simulink model "model"  (R2024a)
settings: Solver=VariableStepAuto  StartTime=0.0  StopTime=10.0  RelTol=1e-3
libraries: dspsigops x11, commdigbbndpm3 x1, commrandsrc3 x1, simulink x1
settings Model: Creator=abc  LastModifiedBy=abc

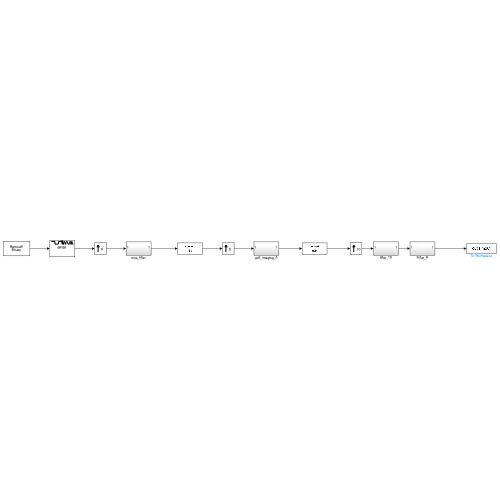
[thumbnail: Simulink's stored preview of the top-level diagram]
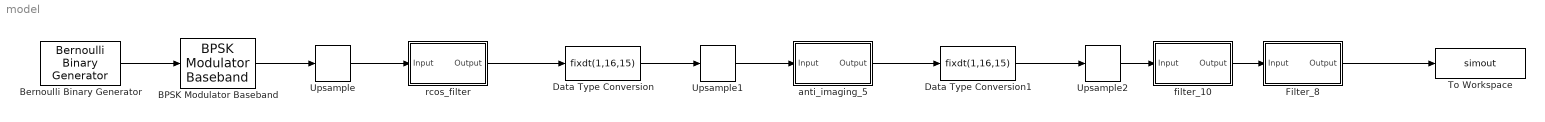
== system model ==
  BPSK Modulator Baseband : commdigbbndpm3/BPSK Modulator Baseband  Ph=0  outDtype=double  outWordLen=16  outUDDataType=sfix(16)  outFracLenMode=Best precision  outFracLen=15  outDataTypeStr=double  outLastDataTypeStr=double
  Bernoulli Binary Generator : commrandsrc3/Bernoulli Binary Generator  ProbabilityOfZero=0.5  SeedSource=Auto  Seed=0  SampleTime=1/400e3  SamplesPerFrame=1  OutputDataType=double  SimulateUsing=Interpreted execution
  Data Type Conversion : DataTypeConversion  OutDataTypeStr=fixdt(1,16,15)  ConvertRealWorld=Stored Integer (SI)  SaturateOnIntegerOverflow=off  RndMeth=Floor
  Data Type Conversion1 : DataTypeConversion  OutDataTypeStr=fixdt(1,16,15)  ConvertRealWorld=Stored Integer (SI)  SaturateOnIntegerOverflow=off  RndMeth=Floor
  Filter_8 : Subsystem  Tag=FilterWizardSubSystem
      settings: ErrorFcn=dspFilterRealizedInBasicElemsAlgLoopErrFcnCallback
  To Workspace : ToWorkspace  VariableName=simout  SampleTime=-1
      settings: Save2DSignal=2-D array (concatenate along first dimension)
  Upsample : dspsigops/Upsample  FactorSource=Dialog parameter  N=9  Nmax=16  phase=0  RateOptions=Allow multirate processing  ic=0  mode=Unused parameter value
  Upsample1 : dspsigops/Upsample  FactorSource=Dialog parameter  N=5  Nmax=16  phase=0  RateOptions=Allow multirate processing  ic=0  mode=Unused parameter value
  Upsample2 : dspsigops/Upsample  FactorSource=Dialog parameter  N=10  Nmax=16  phase=0  RateOptions=Allow multirate processing  ic=0  mode=Unused parameter value
  anti_imaging_5 : Subsystem  Tag=FilterWizardSubSystem
      settings: ErrorFcn=dspFilterRealizedInBasicElemsAlgLoopErrFcnCallback
  filter_10 : Subsystem  Tag=FilterWizardSubSystem
      settings: ErrorFcn=dspFilterRealizedInBasicElemsAlgLoopErrFcnCallback
  rcos_filter : Subsystem  Tag=FilterWizardSubSystem
      settings: ErrorFcn=dspFilterRealizedInBasicElemsAlgLoopErrFcnCallback
  wires:
  Bernoulli Binary Generator/1 -> BPSK Modulator Baseband/1
  BPSK Modulator Baseband/1 -> Upsample/1
  Upsample/1 -> rcos_filter/1(Input)
  rcos_filter/1(Output) -> Data Type Conversion/1
  Data Type Conversion/1 -> Upsample1/1
  Upsample1/1 -> anti_imaging_5/1(Input)
  anti_imaging_5/1(Output) -> Data Type Conversion1/1
  Data Type Conversion1/1 -> Upsample2/1
  Upsample2/1 -> filter_10/1(Input)
  filter_10/1(Output) -> Filter_8/1(Input)
  Filter_8/1(Output) -> To Workspace/1

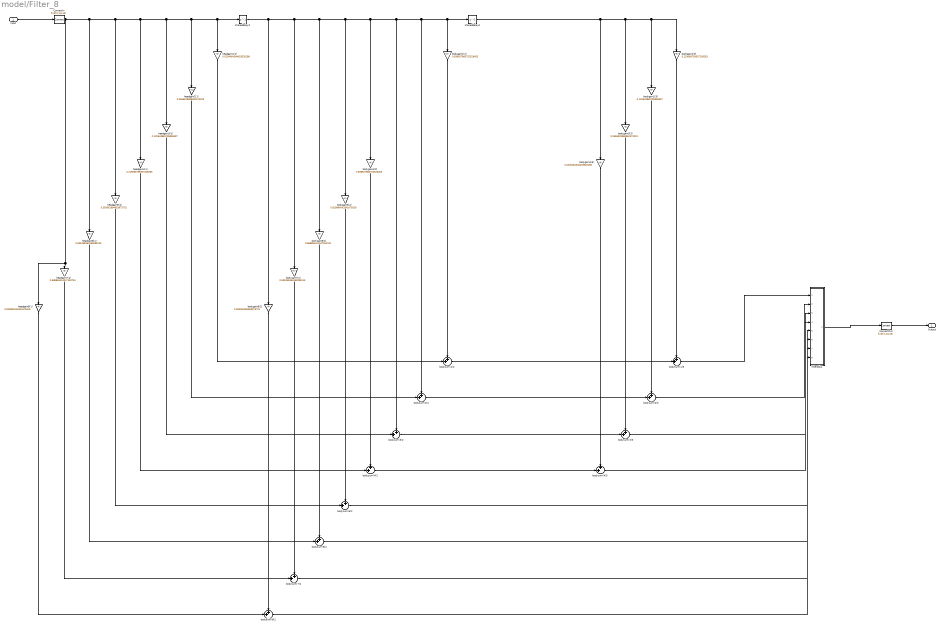
== system model/Filter_8 ==
  Input : Inport
  ConvertIn : DataTypeConversion  OutDataTypeStr=fixdt(1,16,15)  RndMeth=Nearest
  ConvertOut : DataTypeConversion  OutDataTypeStr=fixdt(1,16,15)  RndMeth=Convergent  SaturateOnIntegerOverflow=off
  InterpSys : Subsystem  Tag=FilterWizardInterpolatorCommutator
  bodygain1(2) : Gain  Gain=0.936507860752529453  ParamDataTypeStr=fixdt(1,16,15)  OutDataTypeStr=fixdt(1,31,30)  RndMeth=Convergent
  bodygain1(3) : Gain  Gain=0.219069759307206263  ParamDataTypeStr=fixdt(1,16,15)  OutDataTypeStr=fixdt(1,31,30)  RndMeth=Convergent
  bodygain2(3) : Gain  Gain=0.120643855795995597  ParamDataTypeStr=fixdt(1,16,15)  OutDataTypeStr=fixdt(1,31,30)  RndMeth=Convergent
  bodygain3(3) : Gain  Gain=0.0556329388362373223  ParamDataTypeStr=fixdt(1,16,15)  OutDataTypeStr=fixdt(1,31,30)  RndMeth=Convergent
  bodygain4(2) : Gain  Gain=0.936507860752529453  ParamDataTypeStr=fixdt(1,16,15)  OutDataTypeStr=fixdt(1,31,30)  RndMeth=Convergent
  bodygain4(3) : Gain  Gain=0.0200464348433526188  ParamDataTypeStr=fixdt(1,16,15)  OutDataTypeStr=fixdt(1,31,30)  RndMeth=Convergent
  bodygain5(2) : Gain  Gain=0.819994042841679316  ParamDataTypeStr=fixdt(1,16,15)  OutDataTypeStr=fixdt(1,31,30)  RndMeth=Convergent
  bodygain6(2) : Gain  Gain=0.668884424047150761  ParamDataTypeStr=fixdt(1,16,15)  OutDataTypeStr=fixdt(1,31,30)  RndMeth=Convergent
  bodygain7(2) : Gain  Gain=0.505255361559098115  ParamDataTypeStr=fixdt(1,16,15)  OutDataTypeStr=fixdt(1,31,30)  RndMeth=Convergent
  bodygain8(2) : Gain  Gain=0.350061984653973701  ParamDataTypeStr=fixdt(1,16,15)  OutDataTypeStr=fixdt(1,31,30)  RndMeth=Convergent
  bodysum(1)2 : Sum  Inputs=++|  OutDataTypeStr=fixdt(1,32,30)  AccumDataTypeStr=fixdt(1,32,30)  RndMeth=Convergent
  bodysum(1)3 : Sum  Inputs=++|  OutDataTypeStr=fixdt(1,32,30)  AccumDataTypeStr=fixdt(1,32,30)  RndMeth=Convergent
  bodysum(2)2 : Sum  Inputs=++|  OutDataTypeStr=fixdt(1,32,30)  AccumDataTypeStr=fixdt(1,32,30)  RndMeth=Convergent
  bodysum(2)3 : Sum  Inputs=++|  OutDataTypeStr=fixdt(1,32,30)  AccumDataTypeStr=fixdt(1,32,30)  RndMeth=Convergent
  bodysum(3)2 : Sum  Inputs=++|  OutDataTypeStr=fixdt(1,32,30)  AccumDataTypeStr=fixdt(1,32,30)  RndMeth=Convergent
  bodysum(3)3 : Sum  Inputs=++|  OutDataTypeStr=fixdt(1,32,30)  AccumDataTypeStr=fixdt(1,32,30)  RndMeth=Convergent
  bodysum(4)2 : Sum  Inputs=++|  OutDataTypeStr=fixdt(1,32,30)  AccumDataTypeStr=fixdt(1,32,30)  RndMeth=Convergent
  bodysum(4)3 : Sum  Inputs=++|  OutDataTypeStr=fixdt(1,32,30)  AccumDataTypeStr=fixdt(1,32,30)  RndMeth=Convergent
  bodysum(5)2 : Sum  Inputs=++|  OutDataTypeStr=fixdt(1,32,30)  AccumDataTypeStr=fixdt(1,32,30)  RndMeth=Convergent
  bodysum(6)2 : Sum  Inputs=++|  OutDataTypeStr=fixdt(1,32,30)  AccumDataTypeStr=fixdt(1,32,30)  RndMeth=Convergent
  bodysum(7)2 : Sum  Inputs=++|  OutDataTypeStr=fixdt(1,32,30)  AccumDataTypeStr=fixdt(1,32,30)  RndMeth=Convergent
  bodysum(8)2 : Sum  Inputs=++|  OutDataTypeStr=fixdt(1,32,30)  AccumDataTypeStr=fixdt(1,32,30)  RndMeth=Convergent
  headgain1(1) : Gain  Gain=0.0200464348433526188  ParamDataTypeStr=fixdt(1,16,15)  OutDataTypeStr=fixdt(1,31,30)  RndMeth=Convergent
  headgain2(1) : Gain  Gain=0.0556329388362373223  ParamDataTypeStr=fixdt(1,16,15)  OutDataTypeStr=fixdt(1,31,30)  RndMeth=Convergent
  headgain3(1) : Gain  Gain=0.120643855795995597  ParamDataTypeStr=fixdt(1,16,15)  OutDataTypeStr=fixdt(1,31,30)  RndMeth=Convergent
  headgain4(1) : Gain  Gain=0.219069759307206263  ParamDataTypeStr=fixdt(1,16,15)  OutDataTypeStr=fixdt(1,31,30)  RndMeth=Convergent
  headgain5(1) : Gain  Gain=0.350061984653973701  ParamDataTypeStr=fixdt(1,16,15)  OutDataTypeStr=fixdt(1,31,30)  RndMeth=Convergent
  headgain6(1) : Gain  Gain=0.505255361559098115  ParamDataTypeStr=fixdt(1,16,15)  OutDataTypeStr=fixdt(1,31,30)  RndMeth=Convergent
  headgain7(1) : Gain  Gain=0.668884424047150761  ParamDataTypeStr=fixdt(1,16,15)  OutDataTypeStr=fixdt(1,31,30)  RndMeth=Convergent
  headgain8(1) : Gain  Gain=0.819994042841679316  ParamDataTypeStr=fixdt(1,16,15)  OutDataTypeStr=fixdt(1,31,30)  RndMeth=Convergent
  shareddelay2 : Delay  DelayLength=1  InitialCondition=0
  shareddelay3 : Delay  DelayLength=1  InitialCondition=0
  Output : Outport
  wires:
  headgain1(1)/1 -> bodysum(1)2/2
  headgain2(1)/1 -> bodysum(2)2/2
  headgain3(1)/1 -> bodysum(3)2/2
  headgain4(1)/1 -> bodysum(4)2/2
  headgain5(1)/1 -> bodysum(5)2/2
  headgain6(1)/1 -> bodysum(6)2/2
  headgain7(1)/1 -> bodysum(7)2/2
  headgain8(1)/1 -> bodysum(8)2/2
  Input/1 -> ConvertIn/1
  ConvertIn/1 -> headgain7(1)/1, headgain8(1)/1, headgain1(1)/1, shareddelay2/1, headgain2(1)/1, headgain3(1)/1, headgain4(1)/1, headgain5(1)/1, headgain6(1)/1
  bodygain1(2)/1 -> bodysum(1)2/1
  bodygain4(2)/1 -> bodysum(4)2/1
  bodygain5(2)/1 -> bodysum(5)2/1
  bodygain6(2)/1 -> bodysum(6)2/1
  bodygain7(2)/1 -> bodysum(7)2/1
  bodygain8(2)/1 -> bodysum(8)2/1
  bodysum(1)2/1 -> bodysum(1)3/2
  bodysum(2)2/1 -> bodysum(2)3/2
  bodysum(3)2/1 -> bodysum(3)3/2
  bodysum(4)2/1 -> bodysum(4)3/2
  bodysum(5)2/1 -> InterpSys/5(input5)
  bodysum(6)2/1 -> InterpSys/6(input6)
  bodysum(7)2/1 -> InterpSys/7(input7)
  bodysum(8)2/1 -> InterpSys/8(input8)
  shareddelay2/1 -> bodygain1(2)/1, shareddelay3/1, bodysum(2)2/1, bodysum(3)2/1, bodygain4(2)/1, bodygain5(2)/1, bodygain6(2)/1, bodygain7(2)/1, bodygain8(2)/1
  bodygain1(3)/1 -> bodysum(1)3/1
  bodygain2(3)/1 -> bodysum(2)3/1
  bodygain3(3)/1 -> bodysum(3)3/1
  bodygain4(3)/1 -> bodysum(4)3/1
  bodysum(1)3/1 -> InterpSys/1(input1)
  bodysum(2)3/1 -> InterpSys/2(input2)
  bodysum(3)3/1 -> InterpSys/3(input3)
  bodysum(4)3/1 -> InterpSys/4(input4)
  shareddelay3/1 -> bodygain1(3)/1, bodygain2(3)/1, bodygain3(3)/1, bodygain4(3)/1
  InterpSys/1(output) -> ConvertOut/1
  ConvertOut/1 -> Output/1

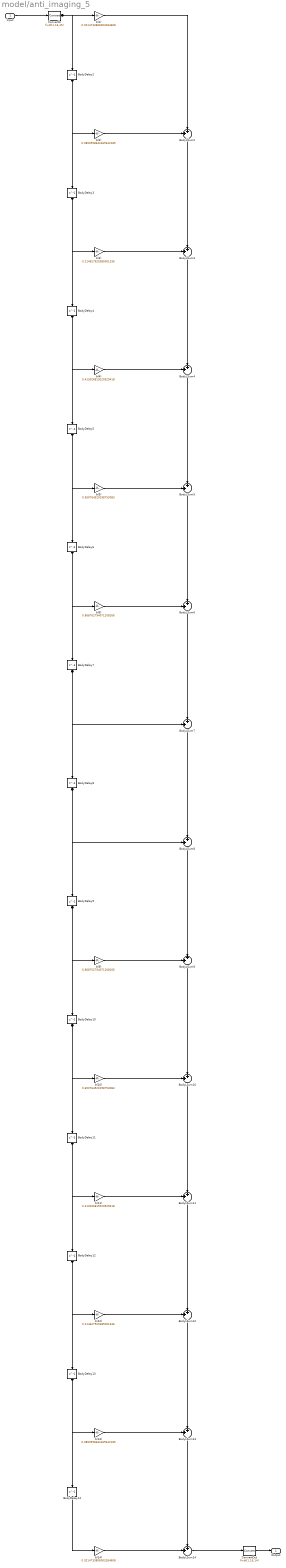
== system model/anti_imaging_5 ==
  Input : Inport
  BodyDelay{2..14} (13 alike) : Delay  DelayLength=1  InitialCondition=0
  BodyLSum{2..14} (13 alike) : Sum  Inputs=++|  OutDataTypeStr=fixdt(1,33,29)  AccumDataTypeStr=fixdt(1,33,29)  RndMeth=Convergent
  ConvertIn : DataTypeConversion  OutDataTypeStr=fixdt(1,16,15)  RndMeth=Nearest
  ConvertOut : DataTypeConversion  OutDataTypeStr=fixdt(1,16,14)  RndMeth=Convergent  SaturateOnIntegerOverflow=off
  b(1) : Gain  Gain=0.0214733806003284608  ParamDataTypeStr=fixdt(1,16,14)  OutDataTypeStr=fixdt(1,31,29)  RndMeth=Convergent
  b(10) : Gain  Gain=0.650764520198753083  ParamDataTypeStr=fixdt(1,16,14)  OutDataTypeStr=fixdt(1,31,29)  RndMeth=Convergent
  b(11) : Gain  Gain=0.413026819220529418  ParamDataTypeStr=fixdt(1,16,14)  OutDataTypeStr=fixdt(1,31,29)  RndMeth=Convergent
  b(12) : Gain  Gain=0.214627920385001336  ParamDataTypeStr=fixdt(1,16,14)  OutDataTypeStr=fixdt(1,31,29)  RndMeth=Convergent
  b(13) : Gain  Gain=0.0850558632469342185  ParamDataTypeStr=fixdt(1,16,14)  OutDataTypeStr=fixdt(1,31,29)  RndMeth=Convergent
  b(14) : Gain  Gain=0.0214733806003284608  ParamDataTypeStr=fixdt(1,16,14)  OutDataTypeStr=fixdt(1,31,29)  RndMeth=Convergent
  b(2) : Gain  Gain=0.0850558632469342185  ParamDataTypeStr=fixdt(1,16,14)  OutDataTypeStr=fixdt(1,31,29)  RndMeth=Convergent
  b(3) : Gain  Gain=0.214627920385001336  ParamDataTypeStr=fixdt(1,16,14)  OutDataTypeStr=fixdt(1,31,29)  RndMeth=Convergent
  b(4) : Gain  Gain=0.413026819220529418  ParamDataTypeStr=fixdt(1,16,14)  OutDataTypeStr=fixdt(1,31,29)  RndMeth=Convergent
  b(5) : Gain  Gain=0.650764520198753083  ParamDataTypeStr=fixdt(1,16,14)  OutDataTypeStr=fixdt(1,31,29)  RndMeth=Convergent
  b(6) : Gain  Gain=0.868762794071208266  ParamDataTypeStr=fixdt(1,16,14)  OutDataTypeStr=fixdt(1,31,29)  RndMeth=Convergent
  b(9) : Gain  Gain=0.868762794071208266  ParamDataTypeStr=fixdt(1,16,14)  OutDataTypeStr=fixdt(1,31,29)  RndMeth=Convergent
  Output : Outport
  wires:
  Input/1 -> ConvertIn/1
  b(1)/1 -> BodyLSum2/2
  ConvertIn/1 -> b(1)/1, BodyDelay2/1
  BodyDelay2/1 -> b(2)/1, BodyDelay3/1
  b(2)/1 -> BodyLSum2/1
  BodyLSum2/1 -> BodyLSum3/2
  BodyDelay3/1 -> b(3)/1, BodyDelay4/1
  b(3)/1 -> BodyLSum3/1
  BodyLSum3/1 -> BodyLSum4/2
  BodyDelay4/1 -> b(4)/1, BodyDelay5/1
  b(4)/1 -> BodyLSum4/1
  BodyLSum4/1 -> BodyLSum5/2
  BodyDelay5/1 -> b(5)/1, BodyDelay6/1
  b(5)/1 -> BodyLSum5/1
  BodyLSum5/1 -> BodyLSum6/2
  BodyDelay6/1 -> b(6)/1, BodyDelay7/1
  b(6)/1 -> BodyLSum6/1
  BodyLSum6/1 -> BodyLSum7/2
  BodyDelay7/1 -> BodyLSum7/1, BodyDelay8/1
  BodyLSum7/1 -> BodyLSum8/2
  BodyDelay8/1 -> BodyLSum8/1, BodyDelay9/1
  BodyLSum8/1 -> BodyLSum9/2
  BodyDelay9/1 -> b(9)/1, BodyDelay10/1
  b(9)/1 -> BodyLSum9/1
  BodyLSum9/1 -> BodyLSum10/2
  BodyDelay10/1 -> b(10)/1, BodyDelay11/1
  b(10)/1 -> BodyLSum10/1
  BodyLSum10/1 -> BodyLSum11/2
  BodyDelay11/1 -> b(11)/1, BodyDelay12/1
  b(11)/1 -> BodyLSum11/1
  BodyLSum11/1 -> BodyLSum12/2
  BodyDelay12/1 -> b(12)/1, BodyDelay13/1
  b(12)/1 -> BodyLSum12/1
  BodyLSum12/1 -> BodyLSum13/2
  BodyDelay13/1 -> b(13)/1, BodyDelay14/1
  b(13)/1 -> BodyLSum13/1
  BodyLSum13/1 -> BodyLSum14/1
  BodyDelay14/1 -> b(14)/1
  b(14)/1 -> BodyLSum14/2
  BodyLSum14/1 -> ConvertOut/1
  ConvertOut/1 -> Output/1

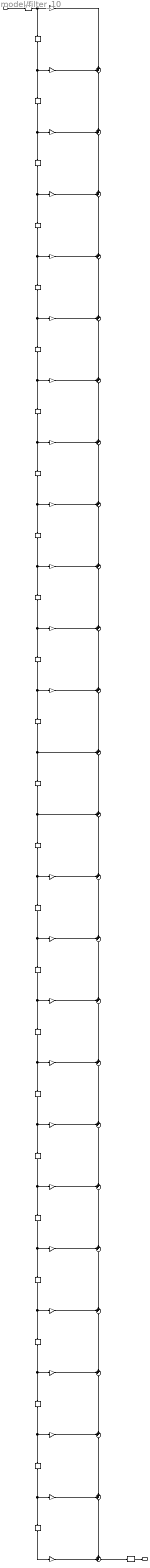
== system model/filter_10 ==
  Input : Inport
  BodyDelay{2..26} (25 alike) : Delay  DelayLength=1  InitialCondition=0
  BodyLSum{2..26} (25 alike) : Sum  Inputs=++|  OutDataTypeStr=fixdt(1,35,30)  AccumDataTypeStr=fixdt(1,35,30)  RndMeth=Convergent
  ConvertIn : DataTypeConversion  OutDataTypeStr=fixdt(1,16,15)  RndMeth=Nearest
  ConvertOut : DataTypeConversion  OutDataTypeStr=fixdt(1,16,15)  RndMeth=Convergent  SaturateOnIntegerOverflow=off
  b(1) : Gain  Gain=0.0154934539007253128  ParamDataTypeStr=fixdt(1,16,15)  OutDataTypeStr=fixdt(1,31,30)  RndMeth=Convergent
  b(10) : Gain  Gain=0.784532005187096648  ParamDataTypeStr=fixdt(1,16,15)  OutDataTypeStr=fixdt(1,31,30)  RndMeth=Convergent
  b(11) : Gain  Gain=0.886548728923319596  ParamDataTypeStr=fixdt(1,16,15)  OutDataTypeStr=fixdt(1,31,30)  RndMeth=Convergent
  b(12) : Gain  Gain=0.960846421505135662  ParamDataTypeStr=fixdt(1,16,15)  OutDataTypeStr=fixdt(1,31,30)  RndMeth=Convergent
  b(15) : Gain  Gain=0.960846421505135662  ParamDataTypeStr=fixdt(1,16,15)  OutDataTypeStr=fixdt(1,31,30)  RndMeth=Convergent
  b(16) : Gain  Gain=0.886548728923319596  ParamDataTypeStr=fixdt(1,16,15)  OutDataTypeStr=fixdt(1,31,30)  RndMeth=Convergent
  b(17) : Gain  Gain=0.784532005187096648  ParamDataTypeStr=fixdt(1,16,15)  OutDataTypeStr=fixdt(1,31,30)  RndMeth=Convergent
  b(18) : Gain  Gain=0.664532684409961938  ParamDataTypeStr=fixdt(1,16,15)  OutDataTypeStr=fixdt(1,31,30)  RndMeth=Convergent
  b(19) : Gain  Gain=0.537212909502194136  ParamDataTypeStr=fixdt(1,16,15)  OutDataTypeStr=fixdt(1,31,30)  RndMeth=Convergent
  b(2) : Gain  Gain=0.0360061265388371618  ParamDataTypeStr=fixdt(1,16,15)  OutDataTypeStr=fixdt(1,31,30)  RndMeth=Convergent
  b(20) : Gain  Gain=0.412761582748364442  ParamDataTypeStr=fixdt(1,16,15)  OutDataTypeStr=fixdt(1,31,30)  RndMeth=Convergent
  b(21) : Gain  Gain=0.299634419816256437  ParamDataTypeStr=fixdt(1,16,15)  OutDataTypeStr=fixdt(1,31,30)  RndMeth=Convergent
  b(22) : Gain  Gain=0.203733323531139293  ParamDataTypeStr=fixdt(1,16,15)  OutDataTypeStr=fixdt(1,31,30)  RndMeth=Convergent
  b(23) : Gain  Gain=0.128056316959141631  ParamDataTypeStr=fixdt(1,16,15)  OutDataTypeStr=fixdt(1,31,30)  RndMeth=Convergent
  b(24) : Gain  Gain=0.0728175851807882912  ParamDataTypeStr=fixdt(1,16,15)  OutDataTypeStr=fixdt(1,31,30)  RndMeth=Convergent
  b(25) : Gain  Gain=0.0360061265388371618  ParamDataTypeStr=fixdt(1,16,15)  OutDataTypeStr=fixdt(1,31,30)  RndMeth=Convergent
  b(26) : Gain  Gain=0.0154934539007253128  ParamDataTypeStr=fixdt(1,16,15)  OutDataTypeStr=fixdt(1,31,30)  RndMeth=Convergent
  b(3) : Gain  Gain=0.0728175851807882912  ParamDataTypeStr=fixdt(1,16,15)  OutDataTypeStr=fixdt(1,31,30)  RndMeth=Convergent
  b(4) : Gain  Gain=0.128056316959141631  ParamDataTypeStr=fixdt(1,16,15)  OutDataTypeStr=fixdt(1,31,30)  RndMeth=Convergent
  b(5) : Gain  Gain=0.203733323531139293  ParamDataTypeStr=fixdt(1,16,15)  OutDataTypeStr=fixdt(1,31,30)  RndMeth=Convergent
  b(6) : Gain  Gain=0.299634419816256437  ParamDataTypeStr=fixdt(1,16,15)  OutDataTypeStr=fixdt(1,31,30)  RndMeth=Convergent
  b(7) : Gain  Gain=0.412761582748364442  ParamDataTypeStr=fixdt(1,16,15)  OutDataTypeStr=fixdt(1,31,30)  RndMeth=Convergent
  b(8) : Gain  Gain=0.537212909502194136  ParamDataTypeStr=fixdt(1,16,15)  OutDataTypeStr=fixdt(1,31,30)  RndMeth=Convergent
  b(9) : Gain  Gain=0.664532684409961938  ParamDataTypeStr=fixdt(1,16,15)  OutDataTypeStr=fixdt(1,31,30)  RndMeth=Convergent
  Output : Outport
  wires:
  Input/1 -> ConvertIn/1
  b(1)/1 -> BodyLSum2/2
  ConvertIn/1 -> b(1)/1, BodyDelay2/1
  BodyDelay2/1 -> b(2)/1, BodyDelay3/1
  b(2)/1 -> BodyLSum2/1
  BodyLSum2/1 -> BodyLSum3/2
  BodyDelay3/1 -> b(3)/1, BodyDelay4/1
  b(3)/1 -> BodyLSum3/1
  BodyLSum3/1 -> BodyLSum4/2
  BodyDelay4/1 -> b(4)/1, BodyDelay5/1
  b(4)/1 -> BodyLSum4/1
  BodyLSum4/1 -> BodyLSum5/2
  BodyDelay5/1 -> b(5)/1, BodyDelay6/1
  b(5)/1 -> BodyLSum5/1
  BodyLSum5/1 -> BodyLSum6/2
  BodyDelay6/1 -> b(6)/1, BodyDelay7/1
  b(6)/1 -> BodyLSum6/1
  BodyLSum6/1 -> BodyLSum7/2
  BodyDelay7/1 -> b(7)/1, BodyDelay8/1
  b(7)/1 -> BodyLSum7/1
  BodyLSum7/1 -> BodyLSum8/2
  BodyDelay8/1 -> b(8)/1, BodyDelay9/1
  b(8)/1 -> BodyLSum8/1
  BodyLSum8/1 -> BodyLSum9/2
  BodyDelay9/1 -> b(9)/1, BodyDelay10/1
  b(9)/1 -> BodyLSum9/1
  BodyLSum9/1 -> BodyLSum10/2
  BodyDelay10/1 -> b(10)/1, BodyDelay11/1
  b(10)/1 -> BodyLSum10/1
  BodyLSum10/1 -> BodyLSum11/2
  BodyDelay11/1 -> b(11)/1, BodyDelay12/1
  b(11)/1 -> BodyLSum11/1
  BodyLSum11/1 -> BodyLSum12/2
  BodyDelay12/1 -> b(12)/1, BodyDelay13/1
  b(12)/1 -> BodyLSum12/1
  BodyLSum12/1 -> BodyLSum13/2
  BodyDelay13/1 -> BodyLSum13/1, BodyDelay14/1
  BodyLSum13/1 -> BodyLSum14/2
  BodyDelay14/1 -> BodyLSum14/1, BodyDelay15/1
  BodyLSum14/1 -> BodyLSum15/2
  BodyDelay15/1 -> b(15)/1, BodyDelay16/1
  b(15)/1 -> BodyLSum15/1
  BodyLSum15/1 -> BodyLSum16/2
  BodyDelay16/1 -> b(16)/1, BodyDelay17/1
  b(16)/1 -> BodyLSum16/1
  BodyLSum16/1 -> BodyLSum17/2
  BodyDelay17/1 -> b(17)/1, BodyDelay18/1
  b(17)/1 -> BodyLSum17/1
  BodyLSum17/1 -> BodyLSum18/2
  BodyDelay18/1 -> b(18)/1, BodyDelay19/1
  b(18)/1 -> BodyLSum18/1
  BodyLSum18/1 -> BodyLSum19/2
  BodyDelay19/1 -> b(19)/1, BodyDelay20/1
  b(19)/1 -> BodyLSum19/1
  BodyLSum19/1 -> BodyLSum20/2
  BodyDelay20/1 -> b(20)/1, BodyDelay21/1
  b(20)/1 -> BodyLSum20/1
  BodyLSum20/1 -> BodyLSum21/2
  BodyDelay21/1 -> b(21)/1, BodyDelay22/1
  b(21)/1 -> BodyLSum21/1
  BodyLSum21/1 -> BodyLSum22/2
  BodyDelay22/1 -> b(22)/1, BodyDelay23/1
  b(22)/1 -> BodyLSum22/1
  BodyLSum22/1 -> BodyLSum23/2
  BodyDelay23/1 -> b(23)/1, BodyDelay24/1
  b(23)/1 -> BodyLSum23/1
  BodyLSum23/1 -> BodyLSum24/2
  BodyDelay24/1 -> b(24)/1, BodyDelay25/1
  b(24)/1 -> BodyLSum24/1
  BodyLSum24/1 -> BodyLSum25/2
  BodyDelay25/1 -> b(25)/1, BodyDelay26/1
  b(25)/1 -> BodyLSum25/1
  BodyLSum25/1 -> BodyLSum26/1
  BodyDelay26/1 -> b(26)/1
  b(26)/1 -> BodyLSum26/2
  BodyLSum26/1 -> ConvertOut/1
  ConvertOut/1 -> Output/1

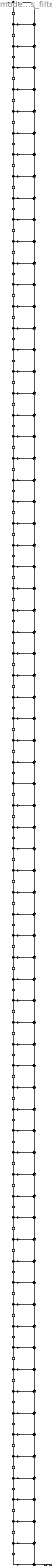
== system model/rcos_filter ==
  Input : Inport
  BodyDelay{2..73} (72 alike) : Delay  DelayLength=1  InitialCondition=0
  BodyLSum{2..73} (72 alike) : Sum  Inputs=++|  OutDataTypeStr=fixdt(1,35,30)  AccumDataTypeStr=fixdt(1,35,30)  RndMeth=Convergent
  ConvertIn : DataTypeConversion  OutDataTypeStr=fixdt(1,16,15)  RndMeth=Nearest
  ConvertOut : DataTypeConversion  OutDataTypeStr=fixdt(1,16,14)  RndMeth=Convergent  SaturateOnIntegerOverflow=off
  b(1) : Gain  Gain=-1.22182503891341904e-17  ParamDataTypeStr=fixdt(1,16,15)  OutDataTypeStr=fixdt(1,31,30)  RndMeth=Convergent
  b(10) : Gain  Gain=2.13059203422986562e-17  ParamDataTypeStr=fixdt(1,16,15)  OutDataTypeStr=fixdt(1,31,30)  RndMeth=Convergent
  b(11) : Gain  Gain=0.021597306460504704  ParamDataTypeStr=fixdt(1,16,15)  OutDataTypeStr=fixdt(1,31,30)  RndMeth=Convergent
  b(12) : Gain  Gain=0.0441571027538437549  ParamDataTypeStr=fixdt(1,16,15)  OutDataTypeStr=fixdt(1,31,30)  RndMeth=Convergent
  b(13) : Gain  Gain=0.0646765061723711676  ParamDataTypeStr=fixdt(1,16,15)  OutDataTypeStr=fixdt(1,31,30)  RndMeth=Convergent
  b(14) : Gain  Gain=0.0799176768301118612  ParamDataTypeStr=fixdt(1,16,15)  OutDataTypeStr=fixdt(1,31,30)  RndMeth=Convergent
  b(15) : Gain  Gain=0.0868181027365576841  ParamDataTypeStr=fixdt(1,16,15)  OutDataTypeStr=fixdt(1,31,30)  RndMeth=Convergent
  b(16) : Gain  Gain=0.0829381759888999509  ParamDataTypeStr=fixdt(1,16,15)  OutDataTypeStr=fixdt(1,31,30)  RndMeth=Convergent
  b(17) : Gain  Gain=0.0668910455890105449  ParamDataTypeStr=fixdt(1,16,15)  OutDataTypeStr=fixdt(1,31,30)  RndMeth=Convergent
  b(18) : Gain  Gain=0.0386959499791306588  ParamDataTypeStr=fixdt(1,16,15)  OutDataTypeStr=fixdt(1,31,30)  RndMeth=Convergent
  b(19) : Gain  Gain=-3.01539353071549505e-17  ParamDataTypeStr=fixdt(1,16,15)  OutDataTypeStr=fixdt(1,31,30)  RndMeth=Convergent
  b(2) : Gain  Gain=-0.00946227947059827962  ParamDataTypeStr=fixdt(1,16,15)  OutDataTypeStr=fixdt(1,31,30)  RndMeth=Convergent
  b(20) : Gain  Gain=-0.0458751609436186536  ParamDataTypeStr=fixdt(1,16,15)  OutDataTypeStr=fixdt(1,31,30)  RndMeth=Convergent
  b(21) : Gain  Gain=-0.0940871562496050223  ParamDataTypeStr=fixdt(1,16,15)  OutDataTypeStr=fixdt(1,31,30)  RndMeth=Convergent
  b(22) : Gain  Gain=-0.138629354352431816  ParamDataTypeStr=fixdt(1,16,15)  OutDataTypeStr=fixdt(1,31,30)  RndMeth=Convergent
  b(23) : Gain  Gain=-0.172866939748332171  ParamDataTypeStr=fixdt(1,16,15)  OutDataTypeStr=fixdt(1,31,30)  RndMeth=Convergent
  b(24) : Gain  Gain=-0.190205163336895938  ParamDataTypeStr=fixdt(1,16,15)  OutDataTypeStr=fixdt(1,31,30)  RndMeth=Convergent
  b(25) : Gain  Gain=-0.184822244508834388  ParamDataTypeStr=fixdt(1,16,15)  OutDataTypeStr=fixdt(1,31,30)  RndMeth=Convergent
  b(26) : Gain  Gain=-0.152386366623032066  ParamDataTypeStr=fixdt(1,16,15)  OutDataTypeStr=fixdt(1,31,30)  RndMeth=Convergent
  b(27) : Gain  Gain=-0.0906723589187520135  ParamDataTypeStr=fixdt(1,16,15)  OutDataTypeStr=fixdt(1,31,30)  RndMeth=Convergent
  b(28) : Gain  Gain=3.66131944315138439e-17  ParamDataTypeStr=fixdt(1,16,15)  OutDataTypeStr=fixdt(1,31,30)  RndMeth=Convergent
  b(29) : Gain  Gain=0.116567855832702696  ParamDataTypeStr=fixdt(1,16,15)  OutDataTypeStr=fixdt(1,31,30)  RndMeth=Convergent
  b(3) : Gain  Gain=-0.0196630498184133598  ParamDataTypeStr=fixdt(1,16,15)  OutDataTypeStr=fixdt(1,31,30)  RndMeth=Convergent
  b(30) : Gain  Gain=0.253304499230267155  ParamDataTypeStr=fixdt(1,16,15)  OutDataTypeStr=fixdt(1,31,30)  RndMeth=Convergent
  b(31) : Gain  Gain=0.402182813135878947  ParamDataTypeStr=fixdt(1,16,15)  OutDataTypeStr=fixdt(1,31,30)  RndMeth=Convergent
  b(32) : Gain  Gain=0.553497404087329614  ParamDataTypeStr=fixdt(1,16,15)  OutDataTypeStr=fixdt(1,31,30)  RndMeth=Convergent
  b(33) : Gain  Gain=0.696689242667723363  ParamDataTypeStr=fixdt(1,16,15)  OutDataTypeStr=fixdt(1,31,30)  RndMeth=Convergent
  b(34) : Gain  Gain=0.821291614576821427  ParamDataTypeStr=fixdt(1,16,15)  OutDataTypeStr=fixdt(1,31,30)  RndMeth=Convergent
  b(35) : Gain  Gain=0.9178999843072434  ParamDataTypeStr=fixdt(1,16,15)  OutDataTypeStr=fixdt(1,31,30)  RndMeth=Convergent
  b(36) : Gain  Gain=0.979063182750591232  ParamDataTypeStr=fixdt(1,16,15)  OutDataTypeStr=fixdt(1,31,30)  RndMeth=Convergent
  b(38) : Gain  Gain=0.979063182750591232  ParamDataTypeStr=fixdt(1,16,15)  OutDataTypeStr=fixdt(1,31,30)  RndMeth=Convergent
  b(39) : Gain  Gain=0.9178999843072434  ParamDataTypeStr=fixdt(1,16,15)  OutDataTypeStr=fixdt(1,31,30)  RndMeth=Convergent
  b(4) : Gain  Gain=-0.0292099363995702542  ParamDataTypeStr=fixdt(1,16,15)  OutDataTypeStr=fixdt(1,31,30)  RndMeth=Convergent
  b(40) : Gain  Gain=0.821291614576821427  ParamDataTypeStr=fixdt(1,16,15)  OutDataTypeStr=fixdt(1,31,30)  RndMeth=Convergent
  b(41) : Gain  Gain=0.696689242667723363  ParamDataTypeStr=fixdt(1,16,15)  OutDataTypeStr=fixdt(1,31,30)  RndMeth=Convergent
  b(42) : Gain  Gain=0.553497404087329614  ParamDataTypeStr=fixdt(1,16,15)  OutDataTypeStr=fixdt(1,31,30)  RndMeth=Convergent
  b(43) : Gain  Gain=0.402182813135878947  ParamDataTypeStr=fixdt(1,16,15)  OutDataTypeStr=fixdt(1,31,30)  RndMeth=Convergent
  b(44) : Gain  Gain=0.253304499230267155  ParamDataTypeStr=fixdt(1,16,15)  OutDataTypeStr=fixdt(1,31,30)  RndMeth=Convergent
  b(45) : Gain  Gain=0.116567855832702696  ParamDataTypeStr=fixdt(1,16,15)  OutDataTypeStr=fixdt(1,31,30)  RndMeth=Convergent
  b(46) : Gain  Gain=3.66131944315138439e-17  ParamDataTypeStr=fixdt(1,16,15)  OutDataTypeStr=fixdt(1,31,30)  RndMeth=Convergent
  b(47) : Gain  Gain=-0.0906723589187520135  ParamDataTypeStr=fixdt(1,16,15)  OutDataTypeStr=fixdt(1,31,30)  RndMeth=Convergent
  b(48) : Gain  Gain=-0.152386366623032066  ParamDataTypeStr=fixdt(1,16,15)  OutDataTypeStr=fixdt(1,31,30)  RndMeth=Convergent
  b(49) : Gain  Gain=-0.184822244508834388  ParamDataTypeStr=fixdt(1,16,15)  OutDataTypeStr=fixdt(1,31,30)  RndMeth=Convergent
  b(5) : Gain  Gain=-0.0365320792686571402  ParamDataTypeStr=fixdt(1,16,15)  OutDataTypeStr=fixdt(1,31,30)  RndMeth=Convergent
  b(50) : Gain  Gain=-0.190205163336895938  ParamDataTypeStr=fixdt(1,16,15)  OutDataTypeStr=fixdt(1,31,30)  RndMeth=Convergent
  b(51) : Gain  Gain=-0.172866939748332171  ParamDataTypeStr=fixdt(1,16,15)  OutDataTypeStr=fixdt(1,31,30)  RndMeth=Convergent
  b(52) : Gain  Gain=-0.138629354352431816  ParamDataTypeStr=fixdt(1,16,15)  OutDataTypeStr=fixdt(1,31,30)  RndMeth=Convergent
  b(53) : Gain  Gain=-0.0940871562496050223  ParamDataTypeStr=fixdt(1,16,15)  OutDataTypeStr=fixdt(1,31,30)  RndMeth=Convergent
  b(54) : Gain  Gain=-0.0458751609436186536  ParamDataTypeStr=fixdt(1,16,15)  OutDataTypeStr=fixdt(1,31,30)  RndMeth=Convergent
  b(55) : Gain  Gain=-3.01539353071549505e-17  ParamDataTypeStr=fixdt(1,16,15)  OutDataTypeStr=fixdt(1,31,30)  RndMeth=Convergent
  b(56) : Gain  Gain=0.0386959499791306588  ParamDataTypeStr=fixdt(1,16,15)  OutDataTypeStr=fixdt(1,31,30)  RndMeth=Convergent
  b(57) : Gain  Gain=0.0668910455890105449  ParamDataTypeStr=fixdt(1,16,15)  OutDataTypeStr=fixdt(1,31,30)  RndMeth=Convergent
  b(58) : Gain  Gain=0.0829381759888999509  ParamDataTypeStr=fixdt(1,16,15)  OutDataTypeStr=fixdt(1,31,30)  RndMeth=Convergent
  b(59) : Gain  Gain=0.0868181027365576841  ParamDataTypeStr=fixdt(1,16,15)  OutDataTypeStr=fixdt(1,31,30)  RndMeth=Convergent
  b(6) : Gain  Gain=-0.0400886182105992597  ParamDataTypeStr=fixdt(1,16,15)  OutDataTypeStr=fixdt(1,31,30)  RndMeth=Convergent
  b(60) : Gain  Gain=0.0799176768301118612  ParamDataTypeStr=fixdt(1,16,15)  OutDataTypeStr=fixdt(1,31,30)  RndMeth=Convergent
  b(61) : Gain  Gain=0.0646765061723711676  ParamDataTypeStr=fixdt(1,16,15)  OutDataTypeStr=fixdt(1,31,30)  RndMeth=Convergent
  b(62) : Gain  Gain=0.0441571027538437549  ParamDataTypeStr=fixdt(1,16,15)  OutDataTypeStr=fixdt(1,31,30)  RndMeth=Convergent
  b(63) : Gain  Gain=0.021597306460504704  ParamDataTypeStr=fixdt(1,16,15)  OutDataTypeStr=fixdt(1,31,30)  RndMeth=Convergent
  b(64) : Gain  Gain=2.13059203422986562e-17  ParamDataTypeStr=fixdt(1,16,15)  OutDataTypeStr=fixdt(1,31,30)  RndMeth=Convergent
  b(65) : Gain  Gain=-0.0181951054212782654  ParamDataTypeStr=fixdt(1,16,15)  OutDataTypeStr=fixdt(1,31,30)  RndMeth=Convergent
  b(66) : Gain  Gain=-0.0313276747222023533  ParamDataTypeStr=fixdt(1,16,15)  OutDataTypeStr=fixdt(1,31,30)  RndMeth=Convergent
  b(67) : Gain  Gain=-0.0386081527320359039  ParamDataTypeStr=fixdt(1,16,15)  OutDataTypeStr=fixdt(1,31,30)  RndMeth=Convergent
  b(68) : Gain  Gain=-0.0400886182105992597  ParamDataTypeStr=fixdt(1,16,15)  OutDataTypeStr=fixdt(1,31,30)  RndMeth=Convergent
  b(69) : Gain  Gain=-0.0365320792686571402  ParamDataTypeStr=fixdt(1,16,15)  OutDataTypeStr=fixdt(1,31,30)  RndMeth=Convergent
  b(7) : Gain  Gain=-0.0386081527320359039  ParamDataTypeStr=fixdt(1,16,15)  OutDataTypeStr=fixdt(1,31,30)  RndMeth=Convergent
  b(70) : Gain  Gain=-0.0292099363995702542  ParamDataTypeStr=fixdt(1,16,15)  OutDataTypeStr=fixdt(1,31,30)  RndMeth=Convergent
  b(71) : Gain  Gain=-0.0196630498184133598  ParamDataTypeStr=fixdt(1,16,15)  OutDataTypeStr=fixdt(1,31,30)  RndMeth=Convergent
  b(72) : Gain  Gain=-0.00946227947059827962  ParamDataTypeStr=fixdt(1,16,15)  OutDataTypeStr=fixdt(1,31,30)  RndMeth=Convergent
  b(73) : Gain  Gain=-1.22182503891341904e-17  ParamDataTypeStr=fixdt(1,16,15)  OutDataTypeStr=fixdt(1,31,30)  RndMeth=Convergent
  b(8) : Gain  Gain=-0.0313276747222023533  ParamDataTypeStr=fixdt(1,16,15)  OutDataTypeStr=fixdt(1,31,30)  RndMeth=Convergent
  b(9) : Gain  Gain=-0.0181951054212782654  ParamDataTypeStr=fixdt(1,16,15)  OutDataTypeStr=fixdt(1,31,30)  RndMeth=Convergent
  Output : Outport
  wires:
  Input/1 -> ConvertIn/1
  b(1)/1 -> BodyLSum2/2
  ConvertIn/1 -> b(1)/1, BodyDelay2/1
  BodyDelay2/1 -> b(2)/1, BodyDelay3/1
  b(2)/1 -> BodyLSum2/1
  BodyLSum2/1 -> BodyLSum3/2
  BodyDelay3/1 -> b(3)/1, BodyDelay4/1
  b(3)/1 -> BodyLSum3/1
  BodyLSum3/1 -> BodyLSum4/2
  BodyDelay4/1 -> b(4)/1, BodyDelay5/1
  b(4)/1 -> BodyLSum4/1
  BodyLSum4/1 -> BodyLSum5/2
  BodyDelay5/1 -> b(5)/1, BodyDelay6/1
  b(5)/1 -> BodyLSum5/1
  BodyLSum5/1 -> BodyLSum6/2
  BodyDelay6/1 -> b(6)/1, BodyDelay7/1
  b(6)/1 -> BodyLSum6/1
  BodyLSum6/1 -> BodyLSum7/2
  BodyDelay7/1 -> b(7)/1, BodyDelay8/1
  b(7)/1 -> BodyLSum7/1
  BodyLSum7/1 -> BodyLSum8/2
  BodyDelay8/1 -> b(8)/1, BodyDelay9/1
  b(8)/1 -> BodyLSum8/1
  BodyLSum8/1 -> BodyLSum9/2
  BodyDelay9/1 -> b(9)/1, BodyDelay10/1
  b(9)/1 -> BodyLSum9/1
  BodyLSum9/1 -> BodyLSum10/2
  BodyDelay10/1 -> b(10)/1, BodyDelay11/1
  b(10)/1 -> BodyLSum10/1
  BodyLSum10/1 -> BodyLSum11/2
  BodyDelay11/1 -> b(11)/1, BodyDelay12/1
  b(11)/1 -> BodyLSum11/1
  BodyLSum11/1 -> BodyLSum12/2
  BodyDelay12/1 -> b(12)/1, BodyDelay13/1
  b(12)/1 -> BodyLSum12/1
  BodyLSum12/1 -> BodyLSum13/2
  BodyDelay13/1 -> b(13)/1, BodyDelay14/1
  b(13)/1 -> BodyLSum13/1
  BodyLSum13/1 -> BodyLSum14/2
  BodyDelay14/1 -> b(14)/1, BodyDelay15/1
  b(14)/1 -> BodyLSum14/1
  BodyLSum14/1 -> BodyLSum15/2
  BodyDelay15/1 -> b(15)/1, BodyDelay16/1
  b(15)/1 -> BodyLSum15/1
  BodyLSum15/1 -> BodyLSum16/2
  BodyDelay16/1 -> b(16)/1, BodyDelay17/1
  b(16)/1 -> BodyLSum16/1
  BodyLSum16/1 -> BodyLSum17/2
  BodyDelay17/1 -> b(17)/1, BodyDelay18/1
  b(17)/1 -> BodyLSum17/1
  BodyLSum17/1 -> BodyLSum18/2
  BodyDelay18/1 -> b(18)/1, BodyDelay19/1
  b(18)/1 -> BodyLSum18/1
  BodyLSum18/1 -> BodyLSum19/2
  BodyDelay19/1 -> b(19)/1, BodyDelay20/1
  b(19)/1 -> BodyLSum19/1
  BodyLSum19/1 -> BodyLSum20/2
  BodyDelay20/1 -> b(20)/1, BodyDelay21/1
  b(20)/1 -> BodyLSum20/1
  BodyLSum20/1 -> BodyLSum21/2
  BodyDelay21/1 -> b(21)/1, BodyDelay22/1
  b(21)/1 -> BodyLSum21/1
  BodyLSum21/1 -> BodyLSum22/2
  BodyDelay22/1 -> b(22)/1, BodyDelay23/1
  b(22)/1 -> BodyLSum22/1
  BodyLSum22/1 -> BodyLSum23/2
  BodyDelay23/1 -> b(23)/1, BodyDelay24/1
  b(23)/1 -> BodyLSum23/1
  BodyLSum23/1 -> BodyLSum24/2
  BodyDelay24/1 -> b(24)/1, BodyDelay25/1
  b(24)/1 -> BodyLSum24/1
  BodyLSum24/1 -> BodyLSum25/2
  BodyDelay25/1 -> b(25)/1, BodyDelay26/1
  b(25)/1 -> BodyLSum25/1
  BodyLSum25/1 -> BodyLSum26/2
  BodyDelay26/1 -> b(26)/1, BodyDelay27/1
  b(26)/1 -> BodyLSum26/1
  BodyLSum26/1 -> BodyLSum27/2
  BodyDelay27/1 -> b(27)/1, BodyDelay28/1
  b(27)/1 -> BodyLSum27/1
  BodyLSum27/1 -> BodyLSum28/2
  BodyDelay28/1 -> b(28)/1, BodyDelay29/1
  b(28)/1 -> BodyLSum28/1
  BodyLSum28/1 -> BodyLSum29/2
  BodyDelay29/1 -> b(29)/1, BodyDelay30/1
  b(29)/1 -> BodyLSum29/1
  BodyLSum29/1 -> BodyLSum30/2
  BodyDelay30/1 -> b(30)/1, BodyDelay31/1
  b(30)/1 -> BodyLSum30/1
  BodyLSum30/1 -> BodyLSum31/2
  BodyDelay31/1 -> b(31)/1, BodyDelay32/1
  b(31)/1 -> BodyLSum31/1
  BodyLSum31/1 -> BodyLSum32/2
  BodyDelay32/1 -> b(32)/1, BodyDelay33/1
  b(32)/1 -> BodyLSum32/1
  BodyLSum32/1 -> BodyLSum33/2
  BodyDelay33/1 -> b(33)/1, BodyDelay34/1
  b(33)/1 -> BodyLSum33/1
  BodyLSum33/1 -> BodyLSum34/2
  BodyDelay34/1 -> b(34)/1, BodyDelay35/1
  b(34)/1 -> BodyLSum34/1
  BodyLSum34/1 -> BodyLSum35/2
  BodyDelay35/1 -> b(35)/1, BodyDelay36/1
  b(35)/1 -> BodyLSum35/1
  BodyLSum35/1 -> BodyLSum36/2
  BodyDelay36/1 -> b(36)/1, BodyDelay37/1
  b(36)/1 -> BodyLSum36/1
  BodyLSum36/1 -> BodyLSum37/2
  BodyDelay37/1 -> BodyLSum37/1, BodyDelay38/1
  BodyLSum37/1 -> BodyLSum38/2
  BodyDelay38/1 -> b(38)/1, BodyDelay39/1
  b(38)/1 -> BodyLSum38/1
  BodyLSum38/1 -> BodyLSum39/2
  BodyDelay39/1 -> b(39)/1, BodyDelay40/1
  b(39)/1 -> BodyLSum39/1
  BodyLSum39/1 -> BodyLSum40/2
  BodyDelay40/1 -> b(40)/1, BodyDelay41/1
  b(40)/1 -> BodyLSum40/1
  BodyLSum40/1 -> BodyLSum41/2
  BodyDelay41/1 -> b(41)/1, BodyDelay42/1
  b(41)/1 -> BodyLSum41/1
  BodyLSum41/1 -> BodyLSum42/2
  BodyDelay42/1 -> b(42)/1, BodyDelay43/1
  b(42)/1 -> BodyLSum42/1
  BodyLSum42/1 -> BodyLSum43/2
  BodyDelay43/1 -> b(43)/1, BodyDelay44/1
  b(43)/1 -> BodyLSum43/1
  BodyLSum43/1 -> BodyLSum44/2
  BodyDelay44/1 -> b(44)/1, BodyDelay45/1
  b(44)/1 -> BodyLSum44/1
  BodyLSum44/1 -> BodyLSum45/2
  BodyDelay45/1 -> b(45)/1, BodyDelay46/1
  b(45)/1 -> BodyLSum45/1
  BodyLSum45/1 -> BodyLSum46/2
  BodyDelay46/1 -> b(46)/1, BodyDelay47/1
  b(46)/1 -> BodyLSum46/1
  BodyLSum46/1 -> BodyLSum47/2
  BodyDelay47/1 -> b(47)/1, BodyDelay48/1
  b(47)/1 -> BodyLSum47/1
  BodyLSum47/1 -> BodyLSum48/2
  BodyDelay48/1 -> b(48)/1, BodyDelay49/1
  b(48)/1 -> BodyLSum48/1
  BodyLSum48/1 -> BodyLSum49/2
  BodyDelay49/1 -> b(49)/1, BodyDelay50/1
  b(49)/1 -> BodyLSum49/1
  BodyLSum49/1 -> BodyLSum50/2
  BodyDelay50/1 -> b(50)/1, BodyDelay51/1
  b(50)/1 -> BodyLSum50/1
  BodyLSum50/1 -> BodyLSum51/2
  BodyDelay51/1 -> b(51)/1, BodyDelay52/1
  b(51)/1 -> BodyLSum51/1
  BodyLSum51/1 -> BodyLSum52/2
  BodyDelay52/1 -> b(52)/1, BodyDelay53/1
  b(52)/1 -> BodyLSum52/1
  BodyLSum52/1 -> BodyLSum53/2
  BodyDelay53/1 -> b(53)/1, BodyDelay54/1
  b(53)/1 -> BodyLSum53/1
  BodyLSum53/1 -> BodyLSum54/2
  BodyDelay54/1 -> b(54)/1, BodyDelay55/1
  b(54)/1 -> BodyLSum54/1
  BodyLSum54/1 -> BodyLSum55/2
  BodyDelay55/1 -> b(55)/1, BodyDelay56/1
  b(55)/1 -> BodyLSum55/1
  BodyLSum55/1 -> BodyLSum56/2
  BodyDelay56/1 -> b(56)/1, BodyDelay57/1
  b(56)/1 -> BodyLSum56/1
  BodyLSum56/1 -> BodyLSum57/2
  BodyDelay57/1 -> b(57)/1, BodyDelay58/1
  b(57)/1 -> BodyLSum57/1
  BodyLSum57/1 -> BodyLSum58/2
  BodyDelay58/1 -> b(58)/1, BodyDelay59/1
  b(58)/1 -> BodyLSum58/1
  BodyLSum58/1 -> BodyLSum59/2
  BodyDelay59/1 -> b(59)/1, BodyDelay60/1
  b(59)/1 -> BodyLSum59/1
  BodyLSum59/1 -> BodyLSum60/2
  BodyDelay60/1 -> b(60)/1, BodyDelay61/1
  b(60)/1 -> BodyLSum60/1
  BodyLSum60/1 -> BodyLSum61/2
  BodyDelay61/1 -> b(61)/1, BodyDelay62/1
  b(61)/1 -> BodyLSum61/1
  BodyLSum61/1 -> BodyLSum62/2
  BodyDelay62/1 -> b(62)/1, BodyDelay63/1
  b(62)/1 -> BodyLSum62/1
  BodyLSum62/1 -> BodyLSum63/2
  BodyDelay63/1 -> b(63)/1, BodyDelay64/1
  b(63)/1 -> BodyLSum63/1
  BodyLSum63/1 -> BodyLSum64/2
  BodyDelay64/1 -> b(64)/1, BodyDelay65/1
  b(64)/1 -> BodyLSum64/1
  BodyLSum64/1 -> BodyLSum65/2
  BodyDelay65/1 -> b(65)/1, BodyDelay66/1
  b(65)/1 -> BodyLSum65/1
  BodyLSum65/1 -> BodyLSum66/2
  BodyDelay66/1 -> b(66)/1, BodyDelay67/1
  b(66)/1 -> BodyLSum66/1
  BodyLSum66/1 -> BodyLSum67/2
  BodyDelay67/1 -> b(67)/1, BodyDelay68/1
  b(67)/1 -> BodyLSum67/1
  BodyLSum67/1 -> BodyLSum68/2
  BodyDelay68/1 -> b(68)/1, BodyDelay69/1
  b(68)/1 -> BodyLSum68/1
  BodyLSum68/1 -> BodyLSum69/2
  BodyDelay69/1 -> b(69)/1, BodyDelay70/1
  b(69)/1 -> BodyLSum69/1
  BodyLSum69/1 -> BodyLSum70/2
  BodyDelay70/1 -> b(70)/1, BodyDelay71/1
  b(70)/1 -> BodyLSum70/1
  BodyLSum70/1 -> BodyLSum71/2
  BodyDelay71/1 -> b(71)/1, BodyDelay72/1
  b(71)/1 -> BodyLSum71/1
  BodyLSum71/1 -> BodyLSum72/2
  BodyDelay72/1 -> b(72)/1, BodyDelay73/1
  b(72)/1 -> BodyLSum72/1
  BodyLSum72/1 -> BodyLSum73/1
  BodyDelay73/1 -> b(73)/1
  b(73)/1 -> BodyLSum73/2
  BodyLSum73/1 -> ConvertOut/1
  ConvertOut/1 -> Output/1

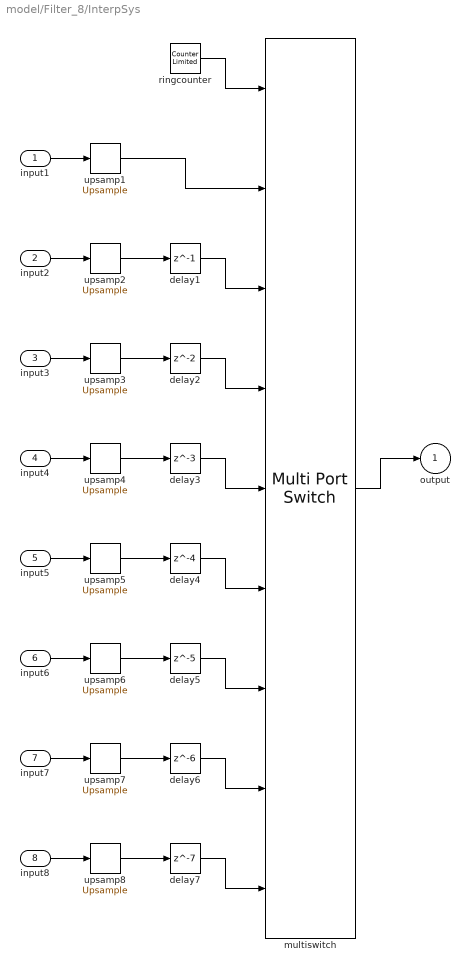
== system model/Filter_8/InterpSys ==
  input1 : Inport
  input2 : Inport  Port=2
  input3 : Inport  Port=3
  input4 : Inport  Port=4
  input5 : Inport  Port=5
  input6 : Inport  Port=6
  input7 : Inport  Port=7
  input8 : Inport  Port=8
  delay1 : Delay  DelayLength=1
  delay2 : Delay
  delay3 : Delay  DelayLength=3
  delay4 : Delay  DelayLength=4
  delay5 : Delay  DelayLength=5
  delay6 : Delay  DelayLength=6
  delay7 : Delay  DelayLength=7
  multiswitch : MultiPortSwitch  DataPortOrder=Zero-based contiguous  Inputs=8  zeroidx=on  InputSameDT=off
  ringcounter : simulink/Sources/Counter Limited  uplimit=7  tsamp=-1
  upsamp{1..8} (8 alike) : dspsigops/Upsample  FactorSource=Dialog parameter  N=8  Nmax=16  phase=0  RateOptions=Allow multirate processing  ic=0  mode=Unused parameter value
  output : Outport
  wires:
  ringcounter/1 -> multiswitch/1
  input1/1 -> upsamp1/1
  upsamp1/1 -> multiswitch/2
  input2/1 -> upsamp2/1
  upsamp2/1 -> delay1/1
  delay1/1 -> multiswitch/3
  input3/1 -> upsamp3/1
  upsamp3/1 -> delay2/1
  delay2/1 -> multiswitch/4
  input4/1 -> upsamp4/1
  upsamp4/1 -> delay3/1
  delay3/1 -> multiswitch/5
  input5/1 -> upsamp5/1
  upsamp5/1 -> delay4/1
  delay4/1 -> multiswitch/6
  input6/1 -> upsamp6/1
  upsamp6/1 -> delay5/1
  delay5/1 -> multiswitch/7
  input7/1 -> upsamp7/1
  upsamp7/1 -> delay6/1
  delay6/1 -> multiswitch/8
  input8/1 -> upsamp8/1
  upsamp8/1 -> delay7/1
  delay7/1 -> multiswitch/9
  multiswitch/1 -> output/1
